simulink model "ssc_1C_Model_NT_MATLABfunc_2RC"  (R2019a)
settings: Solver=VariableStepAuto  StartTime=0  StopTime=0.9623  FixedStep=0.11042  RelTol=1e-4
undefined symbols (not defined in the file): Capacity, tend, tstart
libraries: nesl_utility x4, fl_lib x3
settings Model: OrderedModelArguments=off  Creator=ekonu001  LastModifiedBy=egegs
settings DataIOCC: ExternalInput=t

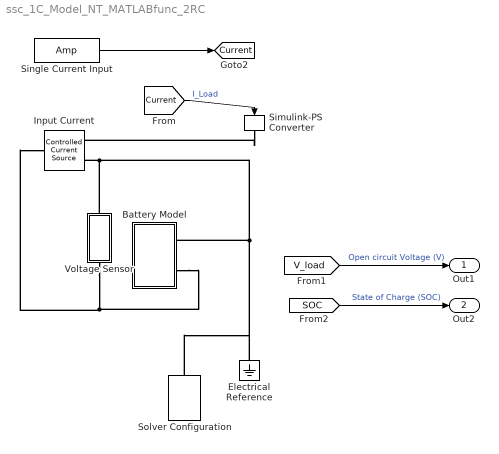
== system ssc_1C_Model_NT_MATLABfunc_2RC ==
  "Battery Model " : Subsystem
  Electrical Reference : fl_lib/Electrical/Electrical Elements/Electrical Reference
  Input Current : fl_lib/Electrical/Electrical Sources/Controlled Current Source
  Simulink-PS Converter : nesl_utility/Simulink-PS Converter  PhysicalDomain=network_engine_domain  SubClassName=ps_input  LeftPortType=input  RightPortType=output  PseudoPeriodic=off  Frequencies=[]  NoiseDistribution=none  NoiseParameters=[]  Unit=A  AffineConversion=off  FilteringAndDerivatives=zero  SimscapeFilterOrder=1  InputFilterTimeConstant=.001  UdotUserProvided=0
  Single Current Input : FromWorkspace  VariableName=Amp  SampleTime=[tend,tstart]
  Solver Configuration : nesl_utility/Solver Configuration  PhysicalDomain=network_engine_domain  SubClassName=solver  LeftPortType=input  RightPortType=generic  Tones=[]  Harmonics=[]  SimulateNoise=off  Profile=off  UseLocalSampling=off  EnableSwitchedLinearOptims=on  FrequencyDomain=off  UseCCode=off  RelTol=0.001  AbsTol=1e-06  MinStep=1e-09  ToWorkspace=off  RevertToSquareIcSolve=off  NumHomotopyIterations=100  PhasorMode=off  PhasorModeNumHarmonics=1  DoDC=off  ResidualTolerance=1e-09  UseLocalSolver=off  LocalSolverChoice=NE_BACKWARD_EULER_ADVANCER  LocalSolverSampleTime=0.001  DoFixedCost=off  MaxNonlinIter=3  MaxModeIter=2  LinearAlgebra=auto  EquationFormulation=NE_TIME_EF  DelaysMemoryBudget=1024  AutomaticFiltering=on  FilteringTimeConstant=0.001  PartitionStorageMethod=AS_NEEDED  PartitionMemoryBudget=1024  PartitionMethod=ROBUST
  Voltage Sensor : Subsystem
      mask Display: disp('V_load')
  Out1 : Outport
  Out2 : Outport  Port=2
  tag scope: Current=global
  wires:
  [Current] -> Simulink-PS Converter/1  "I_Load"
  Single Current Input/1 -> [Current]
  [V_load] -> Out1/1  "Open circuit Voltage (V)"
  [SOC] -> Out2/1  "State of Charge (SOC)"
  connections:
  Solver Configuration/RConn1 -- Electrical Reference/LConn1 -- "Battery Model "/LConn1 -- Voltage Sensor/LConn1 -- Input Current/RConn2
  Voltage Sensor/RConn1 -- "Battery Model "/LConn2 -- Input Current/LConn1
  Simulink-PS Converter/RConn1 -- Input Current/RConn1

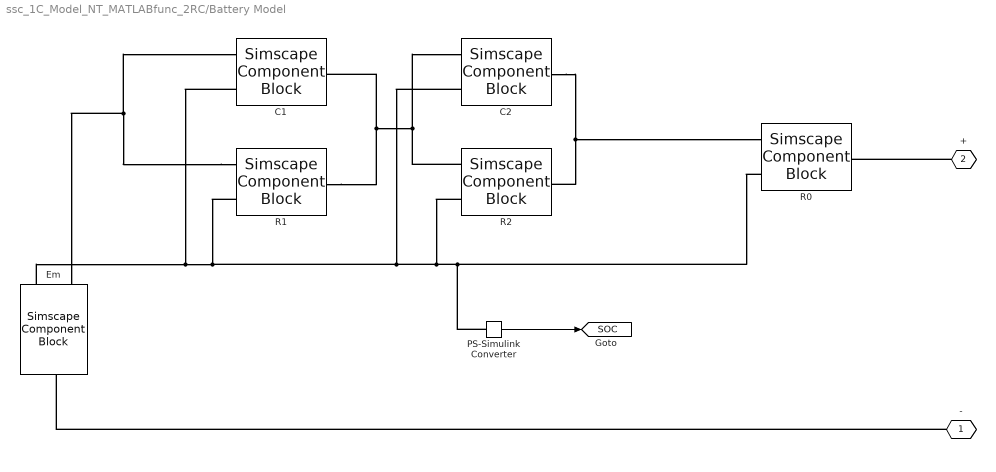
== system ssc_1C_Model_NT_MATLABfunc_2RC/Battery Model  ==
  C1 : SimscapeComponentBlock  SourceFile=LiBatteryElements.C_table_1Temp  ComponentPath=LiBatteryElements.C_table_1Temp  ComponentVariants=LiBatteryElements.C_table_1Temp  ComponentVariantNames=C_table_1Temp  ClassName=C_table_1Temp  SchemaVersion=1  C_Table=C1_LUT F  SOC_Table=SOC_LUT  v0=0 V
      settings: CopyFcn=simscape.engine.sli.internal.componentblockcallback(gcbh,'COPY')  PreCopyFcn=simscape.engine.sli.internal.componentblockcallback(gcbh,'PRECOPY')  PreDeleteFcn=simscape.engine.sli.internal.componentblockcallback(gcbh,'PREDELETE')
      mask Type: C_table_1Temp
  C2 : SimscapeComponentBlock  SourceFile=LiBatteryElements.C_table_1Temp  ComponentPath=LiBatteryElements.C_table_1Temp  ComponentVariants=LiBatteryElements.C_table_1Temp  ComponentVariantNames=C_table_1Temp  ClassName=C_table_1Temp  SchemaVersion=1  C_Table=C2_LUT F  SOC_Table=SOC_LUT  v0=0 V
      settings: CopyFcn=simscape.engine.sli.internal.componentblockcallback(gcbh,'COPY')  PreCopyFcn=simscape.engine.sli.internal.componentblockcallback(gcbh,'PRECOPY')  PreDeleteFcn=simscape.engine.sli.internal.componentblockcallback(gcbh,'PREDELETE')
      mask Type: C_table_1Temp
  Em : SimscapeComponentBlock  SourceFile=LiBatteryElements.Em_table_1Temp  ComponentPath=LiBatteryElements.Em_table_1Temp  ComponentVariants=LiBatteryElements.Em_table_1Temp  ComponentVariantNames=Em_table_1Temp  ClassName=Em_table_1Temp  SchemaVersion=1  Em_Table=Em_LUT V  SOC_Table=SOC_LUT  C=Capacity hr*A  Qinit=Qe_init hr*A
      settings: CopyFcn=simscape.engine.sli.internal.componentblockcallback(gcbh,'COPY')  PreCopyFcn=simscape.engine.sli.internal.componentblockcallback(gcbh,'PRECOPY')  PreDeleteFcn=simscape.engine.sli.internal.componentblockcallback(gcbh,'PREDELETE')
      mask Type: Em_table_1Temp
  PS-Simulink Converter : nesl_utility/PS-Simulink Converter  PhysicalDomain=network_engine_domain  SubClassName=ps_output  LeftPortType=input  RightPortType=output  PseudoPeriodic=off  Frequencies=[]  Unit=1  AffineConversion=off
  R0 : SimscapeComponentBlock  SourceFile=LiBatteryElements.R_table_1Temp  ComponentPath=LiBatteryElements.R_table_1Temp  ComponentVariants=LiBatteryElements.R_table_1Temp  ComponentVariantNames=R_table_1Temp  ClassName=R_table_1Temp  SchemaVersion=1  R_Table=R0_LUT Ohm  SOC_Table=SOC_LUT
      settings: CopyFcn=simscape.engine.sli.internal.componentblockcallback(gcbh,'COPY')  PreCopyFcn=simscape.engine.sli.internal.componentblockcallback(gcbh,'PRECOPY')  PreDeleteFcn=simscape.engine.sli.internal.componentblockcallback(gcbh,'PREDELETE')
      mask Type: R_table_1Temp
  "R1 " : SimscapeComponentBlock  SourceFile=LiBatteryElements.R_table_1Temp  ComponentPath=LiBatteryElements.R_table_1Temp  ComponentVariants=LiBatteryElements.R_table_1Temp  ComponentVariantNames=R_table_1Temp  ClassName=R_table_1Temp  SchemaVersion=1  R_Table=R1_LUT Ohm  SOC_Table=SOC_LUT
      settings: CopyFcn=simscape.engine.sli.internal.componentblockcallback(gcbh,'COPY')  PreCopyFcn=simscape.engine.sli.internal.componentblockcallback(gcbh,'PRECOPY')  PreDeleteFcn=simscape.engine.sli.internal.componentblockcallback(gcbh,'PREDELETE')
      mask Type: R_table_1Temp
  R2 : SimscapeComponentBlock  SourceFile=LiBatteryElements.R_table_1Temp  ComponentPath=LiBatteryElements.R_table_1Temp  ComponentVariants=LiBatteryElements.R_table_1Temp  ComponentVariantNames=R_table_1Temp  ClassName=R_table_1Temp  SchemaVersion=1  R_Table=R2_LUT Ohm  SOC_Table=SOC_LUT
      settings: CopyFcn=simscape.engine.sli.internal.componentblockcallback(gcbh,'COPY')  PreCopyFcn=simscape.engine.sli.internal.componentblockcallback(gcbh,'PRECOPY')  PreDeleteFcn=simscape.engine.sli.internal.componentblockcallback(gcbh,'PREDELETE')
      mask Type: R_table_1Temp
  - : PMIOPort  Tag=PMCPort  Side=Left
  + : PMIOPort  Tag=PMCPort  Port=2  Side=Left
  tag scope: SOC=global
  wires:
  PS-Simulink Converter/1 -> [SOC]
  connections:
  R2/LConn1 -- "R1 "/RConn1 -- C1/RConn1 -- C2/LConn1
  R0/LConn2 -- PS-Simulink Converter/LConn1 -- Em/LConn2 -- C1/LConn2 -- "R1 "/LConn2 -- C2/LConn2 -- R2/LConn2
  R2/RConn1 -- C2/RConn1 -- R0/LConn1
  "R1 "/LConn1 -- Em/LConn1 -- C1/LConn1
  +/RConn1 -- R0/RConn1
  -/RConn1 -- Em/RConn1

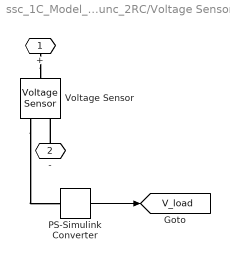
== system ssc_1C_Model_NT_MATLABfunc_2RC/Voltage Sensor ==
  PS-Simulink Converter : nesl_utility/PS-Simulink Converter  PhysicalDomain=network_engine_domain  SubClassName=ps_output  LeftPortType=input  RightPortType=output  PseudoPeriodic=off  Frequencies=[]  Unit=V  AffineConversion=off
  Voltage Sensor : fl_lib/Electrical/Electrical Sensors/Voltage Sensor
  + : PMIOPort  Side=Right
  - : PMIOPort  Port=2  Side=Left
  tag scope: V_load=global
  wires:
  PS-Simulink Converter/1 -> [V_load]
  connections:
  Voltage Sensor/RConn1 -- PS-Simulink Converter/LConn1
  +/RConn1 -- Voltage Sensor/LConn1
  -/RConn1 -- Voltage Sensor/RConn2
